simulink model "TMU5KV400"  (R2018b)
settings: Solver=FixedStepAuto  StartTime=0.0  StopTime=10.0  RelTol=1e-3
PreLoadFcn:
  | load MOTOR_BUS.mat
model workspace (MAT data in the model file):
  Izzm = 1e-05
  Kemf = 0.0041
  Km = 0.0041
  L = 0.0053
  Ra = 0.045
settings Model: Creator=39926  LastModifiedBy=39926

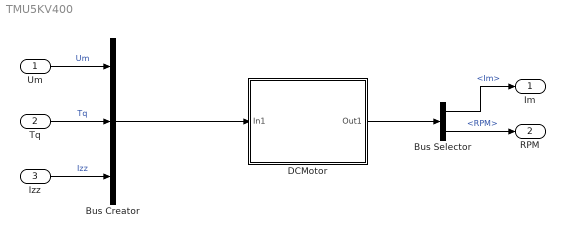
== system TMU5KV400 ==
  Um : Inport  PortDimensions=1
  Tq : Inport  Port=2  PortDimensions=1
  Izz : Inport  Port=3  PortDimensions=1
  Bus Selector : BusSelector  OutputSignals=Im,RPM
  Bus Creator : BusCreator  Inputs=3
  DCMotor : Subsystem  mask{L=0.0000702, Km=0.026228988, Kemf=0.029486916, Imzz=0.00002, Ra=0.0993, I0=0.436382879}
      mask prompts: L "电感值L"; Km "转矩常量Km"; Kemf "反电动势Kemf"; Imzz "转子惯量Imzz"; Ra "电动机内阻Ra"; I0 "空载电流I0"
      mask Display: disp('DCMotor')
  Im : Outport
  RPM : Outport  Port=2
  wires:
  DCMotor/1(Out1) -> Bus Selector/1
  Bus Creator/1 -> DCMotor/1(In1)
  Um/1 -> Bus Creator/1  "Um"
  Tq/1 -> Bus Creator/2  "Tq"
  Izz/1 -> Bus Creator/3  "Izz"
  Bus Selector/1 -> Im/1  "<Im>"
  Bus Selector/2 -> RPM/1  "<RPM>"

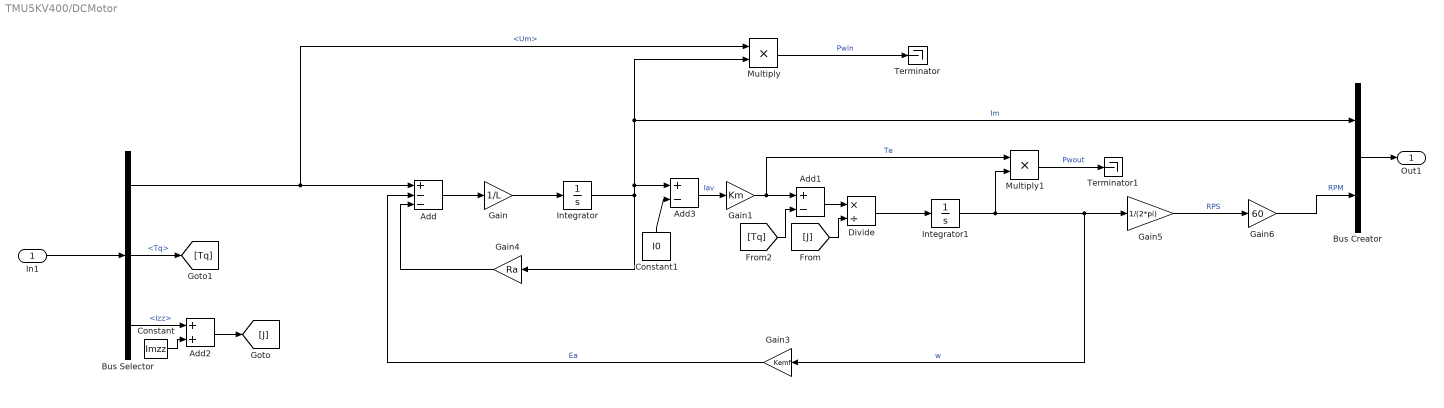
== system TMU5KV400/DCMotor ==
  In1 : Inport
  Add : Sum  Inputs=+--
  Add1 : Sum  Inputs=+-
  Add2 : Sum
  Add3 : Sum  Inputs=+-
  Bus Selector : BusSelector  OutputSignals=Um,Tq,Izz
  Bus Creator : BusCreator  Inputs=2
  Constant : Constant  Value=Imzz
  Constant1 : Constant  Value=I0
  Divide : Product  Inputs=*/
  Gain : Gain  Gain=1/L
  Gain1 : Gain  Gain=Km
  Gain3 : Gain  Gain=Kemf
  Gain4 : Gain  Gain=Ra
  Gain5 : Gain  Gain=1/(2*pi)
  Gain6 : Gain  Gain=60
  Integrator : Integrator  InitialCondition=0.0001
  Integrator1 : Integrator  InitialCondition=0.0001
  Multiply : Product
  Multiply1 : Product
  Terminator : Terminator
  Terminator1 : Terminator
  Out1 : Outport
  wires:
  In1/1 -> Bus Selector/1
  Bus Selector/1 -> Multiply/1, Add/1  "<Um>"
  Add/1 -> Gain/1
  Gain/1 -> Integrator/1
  Integrator/1 -> Add3/1, Multiply/2, Bus Creator/1, Gain4/1  "Im"
  Gain1/1 -> Multiply1/1, Add1/1  "Te"
  Integrator1/1 -> Multiply1/2, Gain3/1, Gain5/1  "w"
  Add1/1 -> Divide/1
  Divide/1 -> Integrator1/1
  Gain3/1 -> Add/2  "Ea"
  Gain4/1 -> Add/3
  Bus Selector/2 -> [Tq]  "<Tq>"
  Bus Selector/3 -> Add2/1  "<Izz>"
  Constant/1 -> Add2/2
  Add2/1 -> [J]
  [J] -> Divide/2
  Multiply/1 -> Terminator/1  "Pwin"
  Multiply1/1 -> Terminator1/1  "Pwout"
  Gain5/1 -> Gain6/1  "RPS"
  Gain6/1 -> Bus Creator/2  "RPM"
  Bus Creator/1 -> Out1/1
  [Tq] -> Add1/2
  Add3/1 -> Gain1/1  "Iav"
  Constant1/1 -> Add3/2
